simulink model "xpcosc"  (Simulink 6.0)
settings: Solver=ode4  StartTime=0.0  StopTime=0.2  FixedStep=0.000250  RelTol=1e-3
settings Model: Creator=mvetsch  LastModifiedBy=ekbas  ExtModeTrigMode=oneshot  ExtModeArmWhenConnect=off  BufferReuse=off
settings DataIOCC: LimitDataPoints=off  SaveState=on  SignalLoggingName=logsOut
settings OptimizationCC: BlockReduction=off  BooleanDataType=off  InlineInvariantSignals=off  OptimizeBlockIOStorage=off  BufferReuse=off  LocalBlockOutputs=off
settings DebuggingCC: CheckExecutionContextPreStartOutputMsg=on  CheckExecutionContextRuntimeOutputMsg=on  SolverPrmCheckMsg=none
settings RTWCC: SystemTargetFile=xpctarget.tlc  TemplateMakefile=xpc_default_tmf  Description=xPC Target  ProcessScript=xpctarget_make_rtw_hook
settings xpcTargetCC: TargetFcnLib=ansi_tfl_tmw.mat  GenFloatMathFcnCalls=ANSI_C  ModelReferenceCompliant=off  LifeSpan=inf
settings SFSimCC: SFSimApplyToAllLibs=on  SFSimBuildMode=Incremental

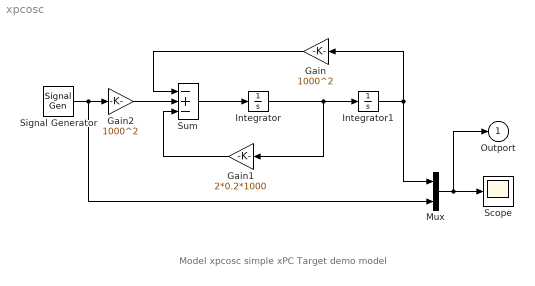
== system xpcosc ==
  note: Model xpcosc
      | simple xPC Target demo model
  Gain : Gain  Orientation=left  Gain=1000^2  SaturateOnIntegerOverflow=on
  Gain1 : Gain  Orientation=left  Gain=2*0.2*1000  SaturateOnIntegerOverflow=on
  Gain2 : Gain  Gain=1000^2  SaturateOnIntegerOverflow=on
  Integrator : Integrator
  Integrator1 : Integrator
  Mux : Mux  Inputs=2
  Scope : Scope
      settings: TickLabels=on  TimeRange=0.200000  YMin=-12  YMax=12  DataFormat=Array
  Signal Generator : SignalGenerator  WaveForm=square  Amplitude=4  Frequency=20
  Sum : Sum  Inputs=-+-  SaturateOnIntegerOverflow=on  InputSameDT=on
  Outport : Outport  InitialOutput=0
  wires:
  Gain2/1 -> Sum/2
  Gain/1 -> Sum/1
  Sum/1 -> Integrator/1
  Integrator/1 -> Integrator1/1, Gain1/1
  Integrator1/1 -> Gain/1, Mux/1
  Gain1/1 -> Sum/3
  Signal Generator/1 -> Gain2/1, Mux/2
  Mux/1 -> Scope/1, Outport/1
